simulink model "test_iir"  (R2018a)
settings: Solver=VariableStepAuto  StartTime=0.0  StopTime=10.0  RelTol=1e-3
libraries: dspsrcs4 x2
settings Model: Creator=hpong  LastModifiedBy=hpong

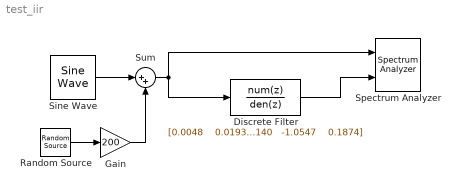
== system test_iir ==
  Discrete Filter : DiscreteFilter  Numerator="[0.0048    0.0193    0.0289    0.0193    0.0048]"  Denominator="[1.0000   -2.3695    2.3140   -1.0547    0.1874]"  InputProcessing=Columns as channels (frame based)  FilterStructure=Direct form I  a0EqualsOne=on
  Gain : Gain  Gain=200
  Random Source : dspsrcs4/Random Source  SrcType=Gaussian  NormMethod=Ziggurat  CltLength=12  MinVal=0  MaxVal=1  MeanVal=0  VarVal=1e-5  RepMode=Specify seed  rawSeed=1  IsInherit=off  SampMode=Discrete  SampTime=1/44100  SampFrame=1024  DataType=Double  OutComplex=Real  OutputFrames=off
  Sine Wave : dspsrcs4/Sine Wave  Amplitude=0.1  Frequency=1000  Phase=0  SampleMode=Discrete  OutComplex=Real  CompMethod=Trigonometric fcn  TableSize=Speed  SampleTime=1/44100  SamplesPerFrame=1024  ResetState=Restart at time zero  OutputFrames=off  dataType=double  wordLen=16  udDataType=sfix(16)  fracBitsMode=Best precision  numFracBits=15  OutDataTypeStr=double  LastOutDataTypeStr=double
  Spectrum Analyzer : SpectrumAnalyzer  NumInputPorts=2
  Sum : Sum  Inputs=|++
  wires:
  Sum/1 -> Discrete Filter/1, Spectrum Analyzer/1
  Discrete Filter/1 -> Spectrum Analyzer/2
  Gain/1 -> Sum/2
  Random Source/1 -> Gain/1
  Sine Wave/1 -> Sum/1
